simulink model "Synchronous_Machine_No_Load_Test"  (R2020a)
settings: Solver=ode5  StartTime=0.0  StopTime=2  RelTol=1e-3
libraries: powerlib x7, powerlib_meascontrol x1
settings Model: Creator=krishna  LastModifiedBy=krishna

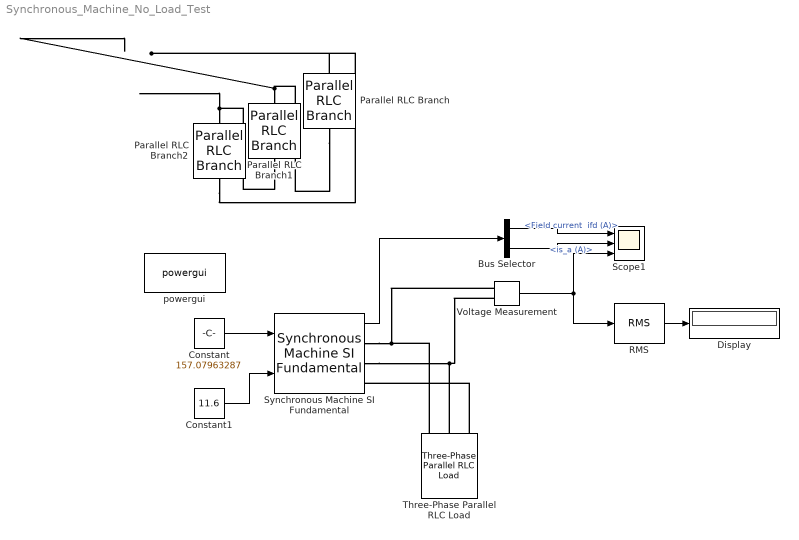
== system Synchronous_Machine_No_Load_Test ==
  Bus Selector : BusSelector  OutputSignals="dq0 components.Field current  ifd (A),Stator current.is_a (A)"
  Constant : Constant  Value=157.07963287
  Constant1 : Constant  Value=11.6
  Display : Display
  Parallel RLC Branch : powerlib/Elements/Parallel RLC Branch  LConnTagsString=a  RConnTagsString=__new0  BranchType=R  Resistance=1e4  Inductance=1e-3  SetiL0=off  InitialCurrent=0  Capacitance=1e-6  Setx0=off  InitialVoltage=0  Measurements=None
  Parallel RLC Branch1 : powerlib/Elements/Parallel RLC Branch  LConnTagsString=a  RConnTagsString=__new0  BranchType=R  Resistance=1e4  Inductance=1e-3  SetiL0=off  InitialCurrent=0  Capacitance=1e-6  Setx0=off  InitialVoltage=0  Measurements=None
  Parallel RLC Branch2 : powerlib/Elements/Parallel RLC Branch  LConnTagsString=a  RConnTagsString=__new0  BranchType=R  Resistance=1e4  Inductance=1e-3  SetiL0=off  InitialCurrent=0  Capacitance=1e-6  Setx0=off  InitialVoltage=0  Measurements=None
  RMS : powerlib_meascontrol/Measurements/RMS  TrueRMS=on  Freq=50  RMSInit=120  Ts=0
  Scope1 : Scope  NumInputPorts=3
  Synchronous Machine SI Fundamental : powerlib/Machines/Synchronous Machine SI Fundamental  PresetModel=01: 50Hz 400V 8.1kVA 1500RPM  MechanicalLoad=Speed w  ShowDetailedParameters=on  RotorType=Salient-pole  Units=SI fundamental parameters  MeasurementBus=off  NominalParameters=[8100 400 50]  Stator=[1.62 0.004527 0.1086 0.05175]  Field=[1.208 0.01132]  Dampers2=[ 0.0664, 1.387e-3, 0.0292, 6.896e-4, 7.907e-3, 2.477e-3]  Dampers1=[3.142 0.007334 4.772 0.01015]  Mechanical=[0.0923 0.009 2]  PolePairs=2  InitialConditions="[ 0  0  0  0  0  0  0  0  70.3192 ]"  SetSaturation=off  Saturation=[695.64,774.7,917.5,1001.6,1082.2,1175.9,1293.6,1430.2,1583.7;9660,10623,12243,13063,13757,14437,15180,15890,16567]  DisplayVfd=off  LoadFlowParameters=[1,0,0,0,0]  TsPowergui=0  TsBlock=-1  IterativeModel=Trapezoidal non iterative  IterativeDiscreteModel=Trapezoidal non iterative  BusType=PV  Pref=0  Qref=0  Qmin=-inf  Qmax=inf  PLF=0  QLF=0
      settings: SourceProductBaseCode=PS
  Three-Phase Parallel RLC Load : powerlib/Elements/Three-Phase Parallel RLC Load  LConnTagsString=A|B|C  Configuration=Delta  NominalVoltage=400  Vabc=[1e3 1e3 1e3]  Vabcp=[1e3 1e3 1e3]  NominalFrequency=50  UnbalancedPower=off  ActivePower=60  InductivePower=30  CapacitivePower=30  Pabc=[10e3 9e3 11e3]  QLabc=[100 90 110]  QCabc=[100 90 110]  Pabcp=[10e3 9e3 11e3]  QLabcp=[100 90 110]  QCabcp=[100 90 110]  Measurements=None  LoadType=constant Z
  Voltage Measurement : powerlib/Measurements/Voltage Measurement  PhasorSimulation=off  OutputType=Complex  PSBequivalent=0
  powergui : powerlib/powergui  Priority=1  SimulationMode=Discrete  SampleTime=5e-6  frequency=60  Iterations=50  frequencyindice=50  Pbase=100e6  ErrMax=1e-4  UnitsV=kV  UnitsW=MW  buscounter=0  FunctionMessages=off  echomessages=off  EnableUseOfTLC=off  CurrentSourceSwitches=off  DisableSnubberDevices=off  DisableRonSwitches=off  DisableVfSwitches=off  DisplayEquations=off  AutomaticDiscreteSolvers=off  SolverType=Tustin/Backward Euler (TBE)  Interpol=off  ExternalGateDelay=off  methode=off  Ts=100  x0status=blocks  SPID=on  SwTol=0  HookPort=off  NonlinearTolerance=1e-4  nMaxIteration=100  ContinueOnMaxIteration=off  RestoreLinks=warning  ResistiveCurrentMeasurement=off  Frange=[0:2:500]  Ylog=off  Xlog=on  ShowGrid=off  save=off  variable=ZData  structure=0  ZoomFFT=off  StartTime=0.0  cycles=1  DisplayStyle=1  fundamental=60  FreqAxis=off  MaxFrequency=1000  frequencyindicesteady=1  RmsSteady=1  display=off
  wires:
  Constant/1 -> Synchronous Machine SI Fundamental/1
  Synchronous Machine SI Fundamental/1 -> Bus Selector/1
  RMS/1 -> Display/1
  Bus Selector/1 -> Scope1/1  "<Field current  ifd (A)>"
  Constant1/1 -> Synchronous Machine SI Fundamental/2
  Voltage Measurement/1 -> Scope1/3, RMS/1
  Bus Selector/2 -> Scope1/2  "<is_a (A)>"
  connections:
  Voltage Measurement/LConn1 -- Three-Phase Parallel RLC Load/LConn1 -- Synchronous Machine SI Fundamental/RConn1
  Parallel RLC Branch1/RConn1 -- Parallel RLC Branch2/LConn1
  Parallel RLC Branch1/LConn1 -- Parallel RLC Branch/RConn1
  Parallel RLC Branch/LConn1 -- Parallel RLC Branch2/RConn1
  Three-Phase Parallel RLC Load/LConn3 -- Synchronous Machine SI Fundamental/RConn3
  Voltage Measurement/LConn2 -- Three-Phase Parallel RLC Load/LConn2 -- Synchronous Machine SI Fundamental/RConn2
